simulink model "daq2_targeting_example"  (R2021b)
settings: Solver=FixedStepDiscrete  StartTime=0.0  StopTime=10.0  RelTol=1e-3
libraries: simulink x17, dsphdlfiltering x4
settings Model: Creator=tcollins  LastModifiedBy=spagadar
settings SolverCC: AlgebraicLoopSolver=TrustRegion
settings DataIOCC: LimitDataPoints=on  SaveOutput=off  SaveTime=off  ReturnWorkspaceOutputs=off
settings OptimizationCC: BlockReduction=off  ConditionallyExecuteInputs=off  DefaultParameterBehavior=Inlined  LifeSpan=inf
settings DebuggingCC: AlgebraicLoopMsg=error  InheritedTsInSrcMsg=none  SingleTaskRateTransMsg=error  AllowSymbolicDim=off  StrictBusMsg=ErrorOnBusTreatedAsVector  SFUnexpectedBacktrackingDiag=warning  SFNoUnconditionalDefaultTransitionDiag=warning  SFExecutionAtInitializationDiag=none  SFMachineParentedDataDiag=warning  ArithmeticOperatorsInVariantConditions=warning
settings HardwareCC: ProdBitPerPointer=32  ProdBitPerSizeT=32  ProdBitPerPtrDiffT=32  ProdLargestAtomicFloat=None  ProdIntDivRoundTo=Undefined  ProdEndianess=Unspecified  ProdWordSize=32  ProdHWDeviceType=ASIC/FPGA->ASIC/FPGA  ProdEqTarget=off
settings SFSimCC: SimUseLocalCustomCode=off  CustomCodeUndefinedFunction=UseInterfaceOnly
settings RTWCC: RTWUseLocalCustomCode=off
settings CodeAppCC: StateflowObjectComments=on
settings GRTTargetCC: TargetLangStandard=C89/C90 (ANSI)
settings ConfigComp: CovScope=ReferencedModels  CovMetricSettings=dw  CovSaveCumulativeToWorkspaceVar=on  CovSaveSingleToWorkspaceVar=on  CovExternalEMLEnable=off  CovSFcnEnable=off

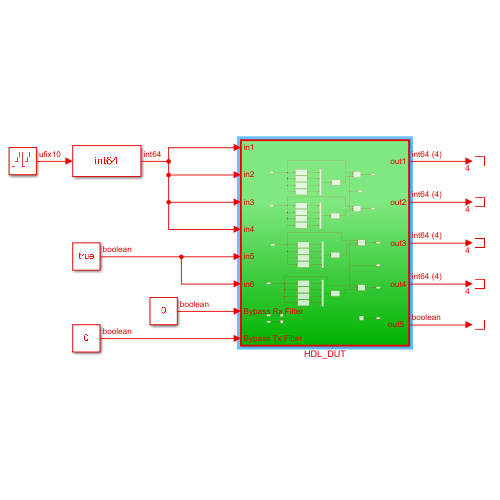
[thumbnail: Simulink's stored preview of the top-level diagram]
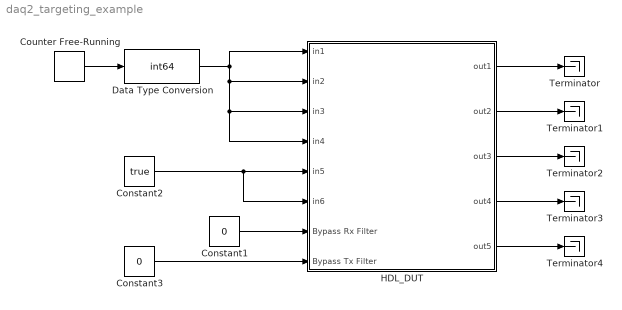
== system daq2_targeting_example ==
  Constant1 : Constant  Value=0  OutDataTypeStr=boolean  SampleTime=-1
  Constant2 : Constant  Value=true  OutDataTypeStr=boolean  SampleTime=-1
  Constant3 : Constant  Value=0  OutDataTypeStr=boolean  SampleTime=-1
  Counter Free-Running : simulink/Sources/Counter Free-Running  NumBits=10  tsamp=1
  Data Type Conversion : DataTypeConversion  OutDataTypeStr=int64
  HDL_DUT : Subsystem  TreatAsAtomicUnit=on
  Terminator{,1..4} (5 alike) : Terminator
  wires:
  Data Type Conversion/1 -> HDL_DUT/4(in4), HDL_DUT/3(in3), HDL_DUT/2(in2), HDL_DUT/1(in1)
  HDL_DUT/4(out4) -> Terminator3/1
  HDL_DUT/3(out3) -> Terminator2/1
  HDL_DUT/2(out2) -> Terminator1/1
  HDL_DUT/1(out1) -> Terminator/1
  Counter Free-Running/1 -> Data Type Conversion/1
  Constant2/1 -> HDL_DUT/6(in6), HDL_DUT/5(in5)
  HDL_DUT/5("out5 ") -> Terminator4/1
  Constant1/1 -> HDL_DUT/7(Bypass Rx Filter)
  Constant3/1 -> HDL_DUT/8(Bypass Tx Filter)

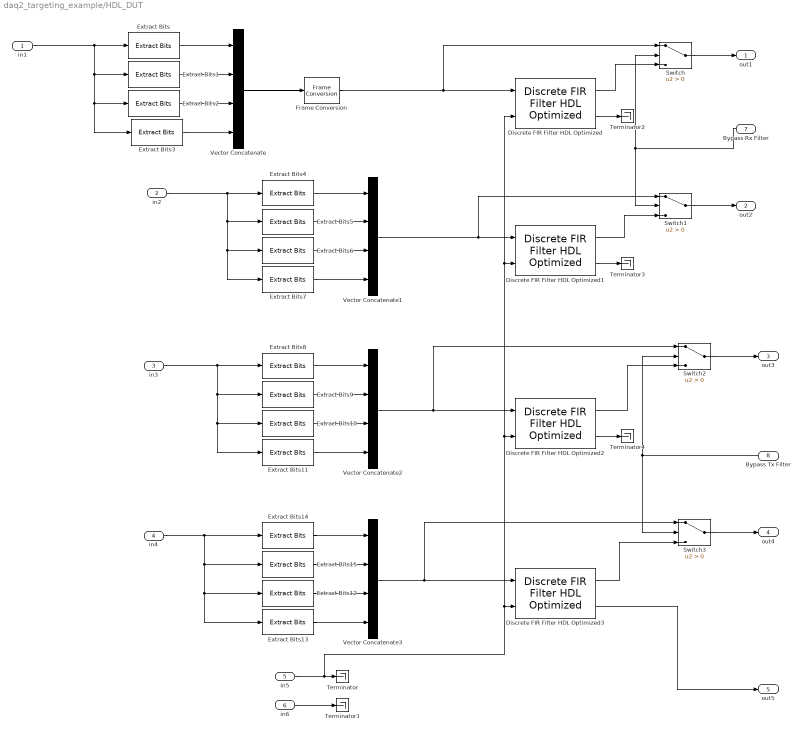
== system daq2_targeting_example/HDL_DUT ==
  in1 : Inport
  in2 : Inport  Port=2
  in3 : Inport  Port=3
  in4 : Inport  Port=4
  in5 : Inport  Port=5
  in6 : Inport  Port=6
  Bypass Rx Filter : Inport  Port=7
  Bypass Tx Filter : Inport  Port=8
  Discrete FIR Filter HDL Optimized{,1..3} (4 alike) : dsphdlfiltering/Discrete FIR Filter HDL Optimized  NumeratorSource=Property  Numerator=[0.125, 0.125, 0.125, 0.125, 0.125, 0.125, 0.125, 0.125]  NumeratorPrototype=[]  FilterStructure=Direct form systolic  SerializationOption=Minimum number of cycles between valid input samples  NumberOfCycles=2  NumberOfMultipliers=2  SimulateUsing=Code generation  roundingMode=Floor  overflowMode=off  CoefficientsDataTypeStr=Inherit: Same word length as input  CoefficientsMin=[]  CoefficientsMax=[]  OutputMin=[]  OutputMax=[]  ResetInputPort=off  HDLGlobalReset=off
      settings: SourceProductBaseCode=DS
  Extract Bits{,4,8,14} (4 alike) : simulink/Logic and Bit Operations/Extract Bits  bitsToExtract=Range of bits  numBits=8  bitIdxRange=[0 15]  outScalingMode=Treat bit field as an integer
  Extract Bits{1,5,9,15} (4 alike) : simulink/Logic and Bit Operations/Extract Bits  bitsToExtract=Range of bits  numBits=8  bitIdxRange=[16 31]  outScalingMode=Treat bit field as an integer
  Extract Bits{2,6,10,12} (4 alike) : simulink/Logic and Bit Operations/Extract Bits  bitsToExtract=Range of bits  numBits=8  bitIdxRange=[32 47]  outScalingMode=Treat bit field as an integer
  Extract Bits{3,7,11,13} (4 alike) : simulink/Logic and Bit Operations/Extract Bits  bitsToExtract=Range of bits  numBits=8  bitIdxRange=[48 63]  outScalingMode=Treat bit field as an integer
  Frame Conversion : FrameConversion  OutFrame=Sample-based
  Switch{,1..3} (4 alike) : Switch  Criteria=u2 > Threshold
  Terminator{,1..4} (5 alike) : Terminator
  Vector Concatenate : Concatenate  NumInputs=4  Mode=Multidimensional array
  Vector Concatenate1 : Concatenate  NumInputs=4
  Vector Concatenate2 : Concatenate  NumInputs=4
  Vector Concatenate3 : Concatenate  NumInputs=4
  out1 : Outport  VectorParamsAs1DForOutWhenUnconnected=off
  out2 : Outport  Port=2  VectorParamsAs1DForOutWhenUnconnected=off
  out3 : Outport  Port=3  VectorParamsAs1DForOutWhenUnconnected=off
  out4 : Outport  Port=4  VectorParamsAs1DForOutWhenUnconnected=off
  "out5 " : Outport  Port=5  VectorParamsAs1DForOutWhenUnconnected=off
  wires:
  in2/1 -> Extract Bits5/1, Extract Bits6/1, Extract Bits7/1, Extract Bits4/1
  in5/1 -> Discrete FIR Filter HDL Optimized3/2, Discrete FIR Filter HDL Optimized2/2, Discrete FIR Filter HDL Optimized1/2, Discrete FIR Filter HDL Optimized/2, Terminator/1
  in6/1 -> Terminator1/1
  in1/1 -> Extract Bits/1, Extract Bits1/1, Extract Bits2/1, Extract Bits3/1
  Switch/1 -> out1/1
  Bypass Rx Filter/1 -> Switch/2, Switch1/2
  Vector Concatenate/1 -> Frame Conversion/1
  Discrete FIR Filter HDL Optimized1/1 -> Switch1/3
  Switch1/1 -> out2/1
  Extract Bits/1 -> Vector Concatenate/1
  Extract Bits1/1 -> Vector Concatenate/2
  Extract Bits2/1 -> Vector Concatenate/3
  Extract Bits3/1 -> Vector Concatenate/4
  Extract Bits4/1 -> Vector Concatenate1/1
  Extract Bits5/1 -> Vector Concatenate1/2
  Extract Bits7/1 -> Vector Concatenate1/4
  Extract Bits6/1 -> Vector Concatenate1/3
  Discrete FIR Filter HDL Optimized2/1 -> Switch2/3
  Switch2/1 -> out3/1
  Extract Bits10/1 -> Vector Concatenate2/3
  Extract Bits11/1 -> Vector Concatenate2/4
  Extract Bits8/1 -> Vector Concatenate2/1
  Extract Bits9/1 -> Vector Concatenate2/2
  in3/1 -> Extract Bits9/1, Extract Bits10/1, Extract Bits11/1, Extract Bits8/1
  Bypass Tx Filter/1 -> Switch2/2, Switch3/2
  Extract Bits15/1 -> Vector Concatenate3/2
  Extract Bits13/1 -> Vector Concatenate3/4
  Extract Bits12/1 -> Vector Concatenate3/3
  Extract Bits14/1 -> Vector Concatenate3/1
  Switch3/1 -> out4/1
  Discrete FIR Filter HDL Optimized3/1 -> Switch3/3
  in4/1 -> Extract Bits12/1, Extract Bits13/1, Extract Bits15/1, Extract Bits14/1
  Vector Concatenate1/1 -> Discrete FIR Filter HDL Optimized1/1, Switch1/1
  Vector Concatenate2/1 -> Discrete FIR Filter HDL Optimized2/1, Switch2/1
  Vector Concatenate3/1 -> Discrete FIR Filter HDL Optimized3/1, Switch3/1
  Discrete FIR Filter HDL Optimized/1 -> Switch/3
  Discrete FIR Filter HDL Optimized/2 -> Terminator2/1
  Discrete FIR Filter HDL Optimized3/2 -> "out5 "/1
  Discrete FIR Filter HDL Optimized1/2 -> Terminator3/1
  Discrete FIR Filter HDL Optimized2/2 -> Terminator4/1
  Frame Conversion/1 -> Switch/1, Discrete FIR Filter HDL Optimized/1
